simulink model "Electrode"  (R2024b)
settings: Solver=ode1  StartTime=0.0  StopTime=10.0  FixedStep=0.0005  RelTol=1e-3
model workspace (MAT data in the model file):
  C = Simulink.Parameter
  C.Value = 1
  C.Complexity = 'real'
  C.Dimensions = [1 1]
  C.DataType = 'auto'
  xi = Simulink.Parameter
  xi.Value = 57.8
  xi.Complexity = 'real'
  xi.Dimensions = [1 1]
  xi.DataType = 'double'
  xj = Simulink.Parameter
  xj.Value = 56.5
  xj.Complexity = 'real'
  xj.Dimensions = [1 1]
  xj.DataType = 'double'
  yi = Simulink.Parameter
  yi.Value = 119.8
  yi.Complexity = 'real'
  yi.Dimensions = [1 1]
  yi.DataType = 'double'
  yj = Simulink.Parameter
  yj.Value = 118
  yj.Complexity = 'real'
  yj.Dimensions = [1 1]
  yj.DataType = 'double'
  zi = Simulink.Parameter
  zi.Value = 0
  zi.Complexity = 'real'
  zi.Dimensions = [1 1]
  zi.DataType = 'double'
  zj = Simulink.Parameter
  zj.Value = 0
  zj.Complexity = 'real'
  zj.Dimensions = [1 1]
  zj.DataType = 'double'
settings Model: DataDictionary=Electrode_dd.sldd  EnableAccessToBaseWorkspace=off  ParameterArgumentNames=C,xi,xj,yi,yj,zi,zj  Creator=wai484  LastModifiedBy=wai484
settings DataIOCC: SaveOutput=off  SignalLogging=off  DSMLogging=off  StreamToWks=off  SaveTime=off  ReturnWorkspaceOutputs=off
settings OptimizationCC: UseDivisionForNetSlopeComputation=UseDivisionForReciprocalsOfIntegersOnly  StateBitsets=on  DataBitsets=on  EfficientFloat2IntCast=on
settings DebuggingCC: SignalInfNanChecking=warning  ReadBeforeWriteMsg=EnableAllAsError  WriteAfterWriteMsg=EnableAllAsError  WriteAfterReadMsg=EnableAllAsError  AlgebraicLoopMsg=error  ArtificialAlgebraicLoopMsg=error  SaveWithDisabledLinksMsg=error  SaveWithParameterizedLinksMsg=error  BlockPriorityViolationMsg=error  TimeAdjustmentMsg=warning  InheritedTsInSrcMsg=error  SingleTaskRateTransMsg=error  TasksWithSamePriorityMsg=error  SigSpecEnsureSampleTimeMsg=error  CheckMatrixSingularityMsg=error  IntegerOverflowMsg=error  ParameterUnderflowMsg=error  ParameterPrecisionLossMsg=error  ParameterTunabilityLossMsg=error  FixptConstUnderflowMsg=error  FixptConstOverflowMsg=error  FixptConstPrecisionLossMsg=error  UnderSpecifiedDataTypeMsg=error  UnnecessaryDatatypeConvMsg=warning  VectorMatrixConversionMsg=error  UnconnectedInputMsg=error  UnconnectedOutputMsg=error  UnconnectedLineMsg=error  SFcnCompatibilityMsg=error  UniqueDataStoreMsg=error  BusObjectLabelMismatch=error  RootOutportRequireBusObject=error  AssertControl=DisableAll  ModelReferenceIOMismatchMessage=error  UnknownTsInhSupMsg=error  ModelReferenceDataLoggingMessage=error  StateNameClashWarn=warning  StrictBusMsg=ErrorOnBusTreatedAsVector  NonBusSignalsTreatedAsBus=error  SFUnusedDataAndEventsDiag=error  SFInvalidInputDataAccessInChartInitDiag=error  SFTransitionOutsideNaturalParentDiag=error  SFUnreachableExecutionPathDiag=error  SFUndirectedBroadcastEventsDiag=error  SFTransitionActionBeforeConditionDiag=error  SFTemporalDelaySmallerThanSampleTimeDiag=error  SFSelfTransitionDiag=error  SFExecutionAtInitializationDiag=error  IntegerSaturationMsg=error  UnderSpecifiedDimensionMsg=error  VariantConditionMismatch=error  InheritVATfromSVC=error  VariantConfigNotUsedByTopModel=error
settings ModelReferenceCC: EnableParallelModelReferenceBuilds=on  PropagateSignalLabelsOutOfModel=off
settings SFSimCC: CompileTimeRecursionLimit=0  EnableRuntimeRecursion=off  MATLABDynamicMemAlloc=off
settings RTWCC: BuildConfiguration=Faster Runs
settings CodeAppCC: ForceParamTrailComments=on  StateflowObjectComments=on  MATLABSourceComments=on
settings GRTTargetCC: UtilityFuncGeneration=Shared location  MatFileLogging=off  SupportNonFinite=off  GenerateSharedConstants=off  OptimizeReductions=on

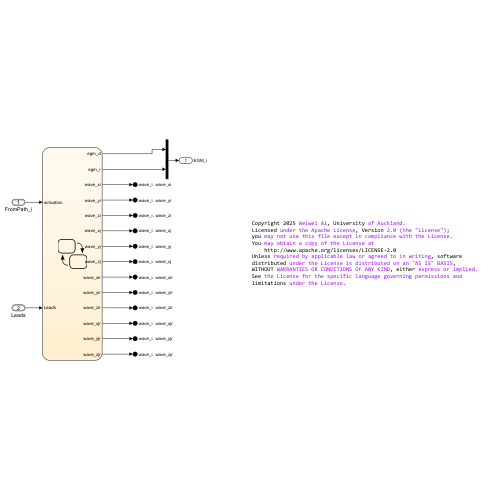
[thumbnail: Simulink's stored preview of the top-level diagram]
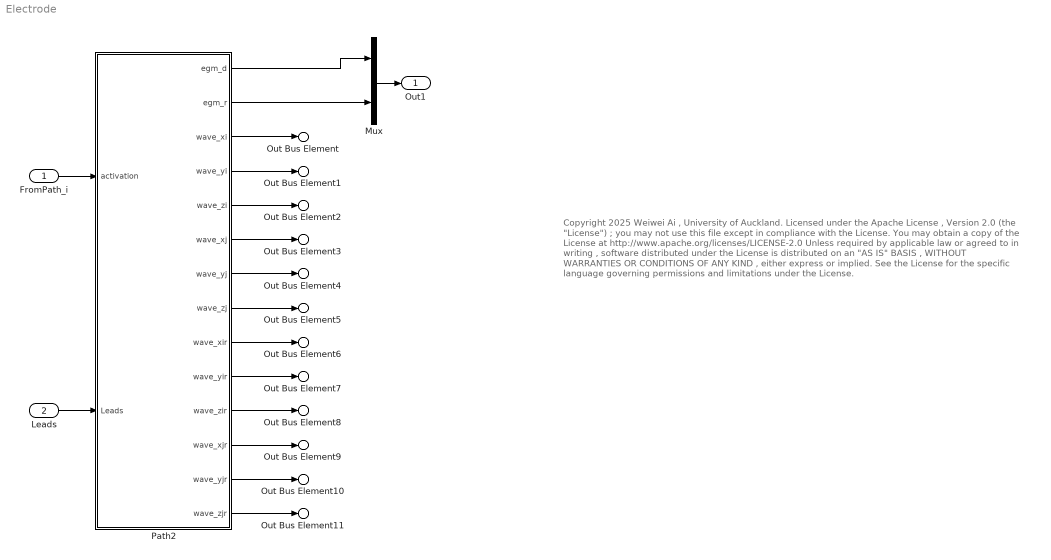
== system Electrode ==
  note: Copyright 2025 Weiwei Ai , University of Auckland.
      | Licensed under the Apache License , Version 2.0 (the "License") ;
      | you may not use this file except in compliance with the License.
      | You may obtain a copy of the License at
      | http://www.apache.org/licenses/LICENSE-2.0
      | Unless required by applicable law or agreed to in writing , software
      | distributed under the License is distributed on an "AS IS" BASIS ,
      | WITHOUT WARRANTIES OR CONDITIONS OF ANY KIND , either express or implied.
      | See the License for the specific language governing permissions and
      | limitations under the License.
  FromPath_i : Inport  OutDataTypeStr=Bus: Activation  BusOutputAsStruct=on
  Leads : Inport  Port=2  OutDataTypeStr=Bus: Lead_group  BusOutputAsStruct=on
  Mux : Mux  Inputs=2
  Path2 : Stateflow chart  TreatAsAtomicUnit=on
  Out1 : Outport  SignalName=EGM_i
  Out Bus Element : Outport  Port=2  PortName=wave_i  Element=wave_xi
  Out Bus Element1 : Outport  Port=2  PortName=wave_i  Element=wave_yi
  Out Bus Element2 : Outport  Port=2  PortName=wave_i  Element=wave_zi
  Out Bus Element3 : Outport  Port=2  PortName=wave_i  Element=wave_xj
  Out Bus Element4 : Outport  Port=2  PortName=wave_i  Element=wave_yj
  Out Bus Element5 : Outport  Port=2  PortName=wave_i  Element=wave_zj
  Out Bus Element6 : Outport  Port=2  PortName=wave_i  Element=wave_xir
  Out Bus Element7 : Outport  Port=2  PortName=wave_i  Element=wave_yir
  Out Bus Element8 : Outport  Port=2  PortName=wave_i  Element=wave_zir
  Out Bus Element9 : Outport  Port=2  PortName=wave_i  Element=wave_xjr
  Out Bus Element10 : Outport  Port=2  PortName=wave_i  Element=wave_yjr
  Out Bus Element11 : Outport  Port=2  PortName=wave_i  Element=wave_zjr
  wires:
  Path2/3(wave_xi) -> Out Bus Element/1
  Path2/4(wave_yi) -> Out Bus Element1/1
  Path2/5(wave_zi) -> Out Bus Element2/1
  Path2/6(wave_xj) -> Out Bus Element3/1
  Path2/7(wave_yj) -> Out Bus Element4/1
  Path2/8(wave_zj) -> Out Bus Element5/1
  Path2/9(wave_xir) -> Out Bus Element6/1
  Path2/10(wave_yir) -> Out Bus Element7/1
  Path2/11(wave_zir) -> Out Bus Element8/1
  Path2/12(wave_xjr) -> Out Bus Element9/1
  Path2/13(wave_yjr) -> Out Bus Element10/1
  Path2/14(wave_zjr) -> Out Bus Element11/1
  FromPath_i/1 -> Path2/1(activation)
  Leads/1 -> Path2/2(Leads)
  Path2/1(egm_d) -> Mux/1
  Path2/2(egm_r) -> Mux/2
  Mux/1 -> Out1/1

== stateflow chart Electrode/Path2 ==
  state EGM1
    state De_wave_i [parallel]
      settings: executionOrder=1
      state Idle
        en:
        egm_d_i=[0 0 0 0]; wave_xi=0; wave_yi=0; wave_zi=0;
      state Active
        du:
        [egm_d_i,wave_xi,wave_yi,wave_zi]  = EGM(activation.cvi,xi,yi,zi,xj,yj,zj,activation.ti,Leads,C);
      EGM1.De_wave_i.Idle -> EGM1.De_wave_i.Active : [activation.ti~=0]
      (default) -> EGM1.De_wave_i.Idle
      EGM1.De_wave_i.Active -> EGM1.De_wave_i.Idle : [activation.ti==0]
    state De_wave_j [parallel]
      settings: executionOrder=2
      state Idle
        en:
        egm_d_j=[0 0 0 0]; wave_xj=0; wave_yj=0; wave_zj=0;
      state Active
        du:
        [egm_d_j,wave_xj,wave_yj, wave_zj]  = EGM(activation.cvj,xj,yj,zj,xi,yi,zi,activation.tj,Leads,C);
      EGM1.De_wave_j.Idle -> EGM1.De_wave_j.Active : [activation.tj~=0]
      (default) -> EGM1.De_wave_j.Idle
      EGM1.De_wave_j.Active -> EGM1.De_wave_j.Idle : [activation.tj==0]
    state Re_wave_i [parallel]
      settings: executionOrder=3
      state Idle
        en:
        egm_r_i=[0 0 0 0]; wave_xir=0; wave_yir=0; wave_zir=0;
      state Active
        du:
        [egm_r_i,wave_xir,wave_yir, wave_zir]  = EGM(activation.cvi,xi,yi,zi,xj,yj,zj,activation.tir,Leads,C);
      EGM1.Re_wave_i.Idle -> EGM1.Re_wave_i.Active : [activation.tir~=0]
      (default) -> EGM1.Re_wave_i.Idle
      EGM1.Re_wave_i.Active -> EGM1.Re_wave_i.Idle : [activation.tir==0]
    state Re_wave_j [parallel]
      settings: executionOrder=4
      state Active
        du:
        [egm_r_j,wave_xjr,wave_yjr, wave_zjr]  = EGM(activation.cvj,xj,yj,zj,xi,yi,zi,activation.tjr,Leads,C);
      state Idle
        en:
        egm_r_j=[0 0 0 0]; wave_xjr=0; wave_yjr=0; wave_zjr=0;
      EGM1.Re_wave_j.Idle -> EGM1.Re_wave_j.Active : [activation.tjr~=0]
      (default) -> EGM1.Re_wave_j.Idle
      EGM1.Re_wave_j.Active -> EGM1.Re_wave_j.Idle : [activation.tjr==0]
    state sum_egm [parallel]
      du:
      egm_r = -egm_r_i.'-egm_r_j.';
      egm_d = egm_d_i.'+egm_d_j.';
      settings: executionOrder=5
  (default) -> EGM1
  data: cv1in function_input; x1in function_input; y1in function_input; z1in function_input; x2in function_input; y2in function_input; z2in function_input; t1in function_input; electrodein function_input; Cin function_input; Potential_d function_output; x11 function_output; y11 function_output; z11 function_output; egm_d output; egm_r output; activation input Bus: Activation; wave_xi output; wave_yi output; wave_zi output; wave_xj output; wave_yj output; wave_zj output; Leads input Bus: Lead_group; wave_xir output; wave_yir output; wave_zir output; wave_xjr output; wave_yjr output; wave_zjr output; xi parameter; yi parameter; zi parameter; xj parameter; yj parameter; zj parameter; C parameter; egm_d_i local; egm_d_j local; egm_r_i local; egm_r_j local
  function [Potential_d,x11,y11,z11]  = EGM(cv1in,x1in,y1in,z1in,x2in,y2in,z2in,t1in,electrodein,Cin):
    | function [Potential_d,x11,y11,z11]  = EGM(cv1in,x1in,y1in,z1in,x2in,y2in,z2in,t1in,electrodein,Cin)
    | %#codegen
    | % ==============================================================
    | %  3D Discrete Moving Dipole Model (Longitudinal + Transversal)
    | %
    | %  The dipole moves from r1 = (x1,y1,z1) to r2 = (x2,y2,z2)
    | %  with speed cv1in.
    | %
    | %  The sensed potential at electrode location r_p is:
    | %
    | %      V = L_scale * (p_long · R)/|R|^3  +  T_scale * (p_trans · R)/|R|^3
    | %
    | %  where:
    | %      D̂     = longitudinal dipole direction (direction of propagation)
    | %      n⊥     = transversal dipole direction (unit vector ⟂ to D̂)
    | %      R      = vector from dipole to electrode
    | %      |R|    = distance from dipole to electrode
    | %
    | % ==============================================================
    | 
    | %% ---------------- Dipole trajectory -------------------------
    | r1 = [x1in, y1in, z1in];
    | r2 = [x2in, y2in, z2in];
    | 
    | D  = r2 - r1;        % displacement vector
    | L  = norm(D);        % path length
    | % if path has zero length, handle gracefully (no motion, dipole fixed at r1)
    | if L == 0
    |     D_hat = [0 0 0]; % Longitudinal dipole (unit vector along motion)
    |     s = 0;
    |     rd = r1;
    | else
    |     D_hat = D / L; % Longitudinal dipole (unit vector along motion)
    |     % dipole position at time t1
    |     s = cv1in * t1in / L;     % fractional position
    |     s = min(max(s,0),1);      % clamp
    |     rd = r1 + s * D;          % dipole coordinates at time t1
    | end
    | 
    | x11 = rd(1);
    | y11 = rd(2);
    | z11 = rd(3);
    | 
    | %% ------------- Electrode group counts ------------------------
    | N=length(fieldnames(electrodein)); % total number of electrodes
    | values=struct2cell(electrodein);
    | Potential_d  = zeros(1,4);
    | 
    | %% ------------------ Dipole vectors ----------------------------
    | 
    | 
    | % --- choose a transversal direction perpendicular to D_hat
    | % We need any vector n_perp such that n_perp · D_hat = 0 and ||n_perp|| = 1
    | if L == 0
    |     % choose arbitrary orthonormal basis
    |     n_perp = [0 0 1];
    | else
    |     % pick a temp vector not parallel to D_hat:
    |     if abs(D_hat(1)) < 0.9
    |         temp = [1 0 0];
    |     else
    |         temp = [0 1 0];
    |     end
    |     n_perp = cross(D_hat, temp);
    |     n_perp_norm = norm(n_perp);
    |     if n_perp_norm < 1e-12
    |         % fallback (very rare): try different temp
    |         temp = [0 0 1];
    |         n_perp = cross(D_hat, temp);
    |         n_perp_norm = norm(n_perp);
    |         if n_perp_norm < 1e-12
    |             % give up and set default
    |             n_perp = [0 0 1];
    |         else
    |             n_perp = n_perp / n_perp_norm;
    |         end
    |     else
    |         n_perp = n_perp / n_perp_norm;
    |     end
    | end
    | 
    | % final longitudinal and transversal dipole directions
    | p_long  = D_hat;
    | p_trans = n_perp;
    | 
    | % weighting of longitudinal and transversal terms
    | L_scale = 1.0;
    | T_scale = 0.1;
    | %% ------------- Loop through all microelectrodes ---------------
    | % small regularizer to avoid infinite values when r==0
    | r_eps = 1e-9 * max(1, L);
    | for j = 1:N
    |     lead_type=values{j}.e_type;
    |     lead_pos=values{j}.e_pos;
    |     rp = [lead_pos.x, lead_pos.y, lead_pos.z];
    |     % vector from dipole to electrode
    |     R = rp - rd;
    |     r = norm(R);
    |     if r < r_eps
    |         r = r_eps;
    |     end
    |     % ----------- Longitudinal dipole potential -----------------
    |     %
    |     %    V_long = (p_long · R) / |R|^3
    |     % -----------------------------------------------------------
    |     V_long = L_scale * dot(p_long, R) / (r^3);
    | 
    |     % ----------- Transversal dipole potential ------------------
    |     %
    |     %    V_trans = (p_trans · R) / |R|^3
    |     %
    |     %   (represents curvature / spread normal to propagation)
    |     % -----------------------------------------------------------
    |     V_trans = T_scale * dot(p_trans, R) / (r^3);
    | 
    |     % Total potential at this microelectrode
    |     EGMall = V_long + V_trans;
    |     switch lead_type
    |         case 1 %'aring'
    |             Potential_d(1)=Potential_d(1)+EGMall * Cin;
    |         case 2 %'atip'
    |             Potential_d(2)=Potential_d(2)+EGMall * Cin;
    |         case 3 %'vring'
    |             Potential_d(3)=Potential_d(3)+EGMall * Cin;
    |         case 4 %'vtip'
    |             Potential_d(4)=Potential_d(4)+EGMall * Cin;
    |         otherwise
    |             error('lead type is unknown')
    | 
    |     end
    | end
    | end
